simulink model "BD_PAR_SS"  (Simulink 10.3)
settings: Solver=ode1  StartTime=0.0  StopTime=max(cyc_mph(:,1))  FixedStep=1  MaxStep=1  RelTol=1e-3  AbsTol=1e-3
undefined symbols (not defined in the file): acc_elec_eff, acc_elec_pwr, acc_mech_eff, amb_tmp, cs_charge_deplete_bool, cs_electric_decel_spd, cs_electric_launch_spd_hi, cs_electric_launch_spd_lo, cs_hi_soc, cs_lo_soc, cs_off_trq_frac, cyc_avg_time, cyc_cargo_mass, cyc_elevation_init, cyc_filter_bool, cyc_grade, cyc_mph, ess_module_num, ess_on, ess_voc, ex_calc, ex_cat_co_frac, ex_cat_ext_cp, ex_cat_ext_emisv, ex_cat_ext_init_tmp, ex_cat_ext_mass, ex_cat_ext_sarea, ex_cat_hc_frac, ex_cat_i2p_th_cond, ex_cat_i2x_emisv, ex_cat_i2x_th_cond, ex_cat_int_cp, ex_cat_int_init_tmp, ex_cat_int_mass, ex_cat_int_sarea, ex_cat_lim, ex_cat_m2i_th_cond, ex_cat_m2i_tmp, ex_cat_m2p_emisv, ex_cat_mon_cp, ex_cat_mon_init_tmp, ex_cat_mon_mass, ex_cat_mon_sarea, ex_cat_monf_sarea, ex_cat_moni_sarea, ex_cat_nox_frac, ex_cat_p2x_th_cond, ex_cat_pcm_ecp, ex_cat_pcm_mass, ex_cat_pcm_tmp, ex_cat_pipe_cp, ex_cat_pipe_emisv, ex_cat_pipe_init_tmp, ex_cat_pipe_mass, ex_cat_pipe_sarea, ex_cat_pm_frac, ex_cat_tmp_range, ex_gas_cp, ex_manif_cp, ex_manif_emisv ... (+73)
libraries: lib_controls x6, lib_vehicle x3, lib_accessory x2, lib_interactive x1, lib_energy_storage x1, lib_fuel_converter x1
(part 3 of 6)

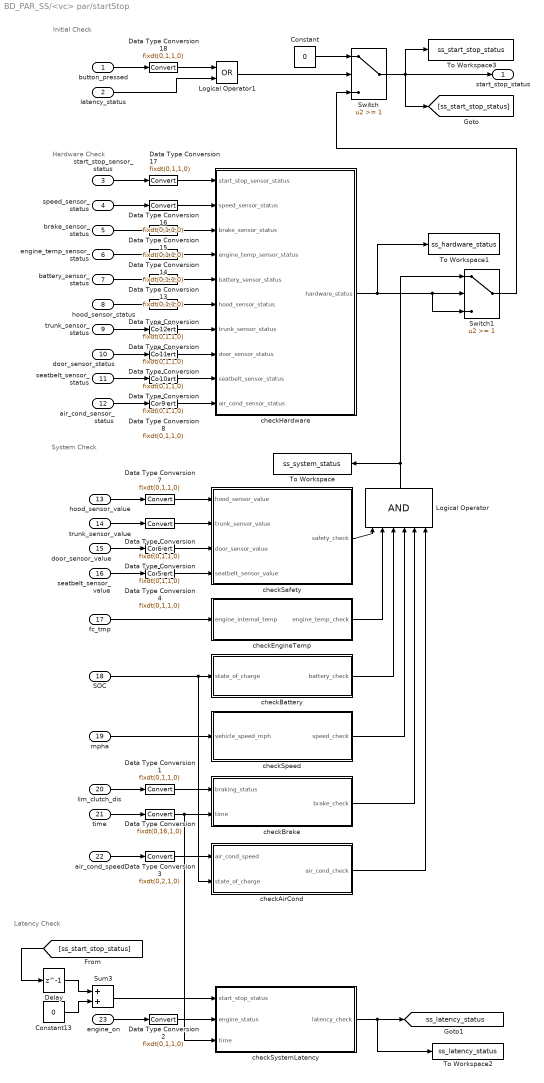
== system BD_PAR_SS/<vc> par/startStop ==
  note: Initial Check
  note: Hardware Check
  note: Latency Check
  note: System Check
  button_pressed : Inport
  latency_status : Inport  Port=2
  start_stop_sensor_status : Inport  Port=3
  speed_sensor_status : Inport  Port=4
  brake_sensor_status : Inport  Port=5
  engine_temp_sensor_status : Inport  Port=6
  battery_sensor_status : Inport  Port=7
  hood_sensor_status : Inport  Port=8
  trunk_sensor_status : Inport  Port=9
  door_sensor_status : Inport  Port=10
  seatbelt_sensor_status : Inport  Port=11
  air_cond_sensor_status : Inport  Port=12
  hood_sensor_value : Inport  Port=13
  trunk_sensor_value : Inport  Port=14
  door_sensor_value : Inport  Port=15
  seatbelt_sensor_value : Inport  Port=16
  fc_tmp : Inport  Port=17
  SOC : Inport  Port=18
  mpha : Inport  Port=19
  lim_clutch_dis : Inport  Port=20
  time : Inport  Port=21
  air_cond_speed : Inport  Port=22
  engine_on : Inport  Port=23
  Constant : Constant  Value=0  OutDataTypeStr=fixdt(0,1,1,0)
  Constant13 : Constant  Value=0  OutDataTypeStr=fixdt(0,1,1,0)
  Data Type Conversion : DataTypeConversion  OutDataTypeStr=fixdt(0,16,1,0)
  Data Type Conversion{1..2,4..18} (17 alike) : DataTypeConversion  OutDataTypeStr=fixdt(0,1,1,0)
  Data Type Conversion3 : DataTypeConversion  OutDataTypeStr=fixdt(0,2,1,0)
  Delay : Delay  DelayLength=1  InitialCondition=0
  Logical Operator : Logic  Inputs=6  AllPortsSameDT=off  OutDataTypeStr=fixdt(0,1,1,0)
  Logical Operator1 : Logic  Operator=OR  AllPortsSameDT=off  OutDataTypeStr=fixdt(0,1,1,0)
  Sum3 : Sum  OutDataTypeStr=fixdt(0,1,1,0)
  Switch : Switch  Threshold=1  OutDataTypeStr=fixdt(0,1,1,0)
  Switch1 : Switch  Threshold=1  OutDataTypeStr=fixdt(0,1,1,0)
  To Workspace : ToWorkspace  VariableName=ss_system_status  SampleTime=-1
  To Workspace1 : ToWorkspace  VariableName=ss_hardware_status  SampleTime=-1
  To Workspace2 : ToWorkspace  VariableName=ss_latency_status  SampleTime=-1
  To Workspace3 : ToWorkspace  VariableName=ss_start_stop_status  SampleTime=-1
  checkAirCond : Subsystem
  checkBattery : Subsystem
  checkBrake : Subsystem
  checkEngineTemp : Subsystem
  checkHardware : Subsystem
  checkSafety : Subsystem
  checkSpeed : Subsystem
  checkSystemLatency : Subsystem
  start_stop_status : Outport
  tag scope: ss_latency_status=global
  wires:
  engine_temp_sensor_status/1 -> Data Type Conversion14/1
  speed_sensor_status/1 -> Data Type Conversion16/1
  Switch/1 -> [ss_start_stop_status], start_stop_status/1, To Workspace3/1
  trunk_sensor_status/1 -> Data Type Conversion11/1
  hood_sensor_status/1 -> Data Type Conversion12/1
  brake_sensor_status/1 -> Data Type Conversion15/1
  battery_sensor_status/1 -> Data Type Conversion13/1
  door_sensor_status/1 -> Data Type Conversion10/1
  seatbelt_sensor_status/1 -> Data Type Conversion9/1
  air_cond_sensor_status/1 -> Data Type Conversion8/1
  button_pressed/1 -> Data Type Conversion18/1
  latency_status/1 -> Logical Operator1/2
  Logical Operator1/1 -> Switch/2
  start_stop_sensor_status/1 -> Data Type Conversion17/1
  checkHardware/1(hardware_status) -> Switch1/2, Switch1/3, To Workspace1/1
  hood_sensor_value/1 -> Data Type Conversion7/1
  trunk_sensor_value/1 -> Data Type Conversion6/1
  door_sensor_value/1 -> Data Type Conversion5/1
  seatbelt_sensor_value/1 -> Data Type Conversion4/1
  fc_tmp/1 -> checkEngineTemp/1(engine_internal_temp)
  SOC/1 -> checkAirCond/2(state_of_charge), checkBattery/1(state_of_charge)
  mpha/1 -> checkSpeed/1(vehicle_speed_mph)
  air_cond_speed/1 -> Data Type Conversion3/1
  time/1 -> Data Type Conversion/1
  lim_clutch_dis/1 -> Data Type Conversion1/1
  checkSafety/1(safety_check) -> Logical Operator/1
  checkEngineTemp/1(engine_temp_check) -> Logical Operator/2
  checkBattery/1(battery_check) -> Logical Operator/3
  checkSpeed/1(speed_check) -> Logical Operator/4
  checkBrake/1(brake_check) -> Logical Operator/5
  checkAirCond/1(air_cond_check) -> Logical Operator/6
  Logical Operator/1 -> Switch1/1, To Workspace/1
  Constant/1 -> Switch/1
  Switch1/1 -> Switch/3
  engine_on/1 -> Data Type Conversion2/1
  checkSystemLatency/1(latency_check) -> [ss_latency_status], To Workspace2/1
  Sum3/1 -> checkSystemLatency/1(start_stop_status)
  [ss_start_stop_status] -> Delay/1
  Data Type Conversion/1 -> checkSystemLatency/3(time), checkBrake/2(time)
  Data Type Conversion1/1 -> checkBrake/1(braking_status)
  Data Type Conversion2/1 -> checkSystemLatency/2(engine_status)
  Data Type Conversion3/1 -> checkAirCond/1(air_cond_speed)
  Constant13/1 -> Sum3/2
  Delay/1 -> Sum3/1
  Data Type Conversion4/1 -> checkSafety/4(seatbelt_sensor_value)
  Data Type Conversion5/1 -> checkSafety/3(door_sensor_value)
  Data Type Conversion6/1 -> checkSafety/2(trunk_sensor_value)
  Data Type Conversion7/1 -> checkSafety/1(hood_sensor_value)
  Data Type Conversion8/1 -> checkHardware/10(air_cond_sensor_status)
  Data Type Conversion9/1 -> checkHardware/9(seatbelt_sensor_status)
  Data Type Conversion10/1 -> checkHardware/8(door_sensor_status)
  Data Type Conversion11/1 -> checkHardware/7(trunk_sensor_status)
  Data Type Conversion14/1 -> checkHardware/4(engine_temp_sensor_status)
  Data Type Conversion15/1 -> checkHardware/3(brake_sensor_status)
  Data Type Conversion13/1 -> checkHardware/5(battery_sensor_status)
  Data Type Conversion12/1 -> checkHardware/6(hood_sensor_status)
  Data Type Conversion16/1 -> checkHardware/2(speed_sensor_status)
  Data Type Conversion17/1 -> checkHardware/1(start_stop_sensor_status)
  Data Type Conversion18/1 -> Logical Operator1/1

== system BD_PAR_SS/NOTES/NOTES ==
  note: ADVISOR 2.0.2 10/7/98
      | Copyright 1998-2003  MRI, NREL.
      | All rights reserved
      |
      |  Notice:  This computer software was
      |  prepared by NREL/MRI, and hereinafter the Contractor,
      | under Contract No. DE-AC36-83CH10093 with
      | the Department of Energy (DOE).  All rights
      | in the computer software are reserved by DOE
      | on behalf of the United States Government and
      | the Contractor as provided in the contract.
      | You are authorized to use this computer software
      | for Governmental purposes but it is not to be
      | released or distributed to the public.  NEITHER
      | THE GOVERNMENT NOR THE CONTRACTOR MAKES ANY
      | WARRANTY, EXPRESS OR IMPLIED, OR ASSUMES ANY
      | LIABILITY FOR THE USE OF THIS SOFTWARE.
      | This notice including this sentence must
      | appear on any copies of this computer software.

== system BD_PAR_SS/clutch <cl>/help ==

== system BD_PAR_SS/drive cycle <cyc>/Block NOTES ==
  note: This block determines the speed required of the vehicle.  If cyc_filter_bool
      | is true, a centered-in-time average of the trace, with backlash, is required of
      | the vehicle.  This may be useful to smooth out jumps in the trace.  Otherwise,
      | the trace, exactly as published, is required of the vehicle.
      | This block also determines the roadway grade of the cycle and the
      | elevation as a function of the distance travelelled

== system BD_PAR_SS/drive cycle <cyc>/ambient pressure calc (atm) ==
  elevation : Inport
  Gain1 : Gain  Gain=-1  SaturateOnIntegerOverflow=on  OutDataTypeStr=Inherit: Same as input  ParamDataTypeStr=Inherit: Same as input
  Height Scale Factor (1/m) : Constant  Value=1.16546e-4
  Math Function : Math  SignedPower=on  SaturateOnIntegerOverflow=on
  Product9 : Product  InputSameDT=on  RndMeth=Zero  SaturateOnIntegerOverflow=on  OutDataTypeStr=Inherit: Same as first input
  Out1 : Outport
  wires:
  Math Function/1 -> Out1/1
  Height Scale Factor (1/m)/1 -> Product9/2
  Gain1/1 -> Product9/1
  elevation/1 -> Gain1/1
  Product9/1 -> Math Function/1

== system BD_PAR_SS/drive cycle <cyc>/distance travelled (m) ==
  Block NOTES : Subsystem
      mask Display: disp('Block\nNOTES')
  Integrator : Integrator
  mph-->m/s : Gain  Gain=0.447  SaturateOnIntegerOverflow=on  OutDataTypeStr=Inherit: Same as input  ParamDataTypeStr=Inherit: Same as input
  Out1 : Outport  InitialOutput=0
  wires:
  mph-->m/s/1 -> Integrator/1
  [mpha] -> mph-->m/s/1
  Integrator/1 -> Out1/1

== system BD_PAR_SS/drive cycle <cyc>/repeated cycle grade vs. distance ==
  distance travelled (m) : Inport
  Fcn1 : Fcn  Expr=rem(u[1],period)
  Look-Up Table : Lookup  InputValues=t  Table=y  SaturateOnIntegerOverflow=on
  out_1 : Outport  InitialOutput=0
  wires:
  Look-Up Table/1 -> out_1/1
  Fcn1/1 -> Look-Up Table/1
  distance travelled (m)/1 -> Fcn1/1

== system BD_PAR_SS/drive cycle <cyc>/repeated cycle speed vs. time ==
  Clock : Clock
  Fcn1 : Fcn  Expr=rem(u[1],period)
  Look-Up Table : Lookup  InputValues=t  Table=y  SaturateOnIntegerOverflow=on
  out_1 : Outport  InitialOutput=0
  wires:
  Look-Up Table/1 -> out_1/1
  Clock/1 -> Fcn1/1
  Fcn1/1 -> Look-Up Table/1

== system BD_PAR_SS/drive cycle <cyc>/repeated cycle vehicle cargo mass vs. distance ==
  distance travelled (m) : Inport
  Fcn1 : Fcn  Expr=rem(u[1],period)
  Look-Up Table : Lookup  InputValues=t  Table=y  SaturateOnIntegerOverflow=on
  out_1 : Outport  InitialOutput=0
  wires:
  Look-Up Table/1 -> out_1/1
  Fcn1/1 -> Look-Up Table/1
  distance travelled (m)/1 -> Fcn1/1

== system BD_PAR_SS/drive cycle <cyc>/super-smooth, no-lag trace ==
  Subsystem : Subsystem  mask(Running Average){n=avgtime}
      mask prompts: n "Averaging Time (s)"
      mask help: Running Average
      mask Help: Output is the average of the last (Averaging Time) seconds of input.
      mask Display: disp('Running\nAverage')
  repeated cycle : Subsystem
  out_1 : Outport  InitialOutput=0
  wires:
  repeated cycle/1(out_1) -> Subsystem/1(in_1)
  Subsystem/1(out_1) -> out_1/1

== system BD_PAR_SS/electric acc loads <acc>/Electrical Accessory Loads v2 <acc> ==
  note: Data Logging
  note: Backward-Forward Models
  note: INTERFACE
  "requested electrical Power, out to the driveline (W)" : Inport
  achieved power in from power source (W) : Inport  Port=2
  on/off : Inport  Port=3
  Accessory SDO : Subsystem
  Block NOTES : Subsystem
      mask Display: disp('Block\nNOTES')
  Mux3 : Mux  Inputs=3
  backward model : Subsystem
  forward model : Subsystem
  memory : Memory  InitialCondition=acc_elec_pwr
  "requested electrical Power, in from the power source (W)" : Outport
  "achieved electrical Power, out to the driveline (W)" : Outport  Port=2
  tag scope: acc_elec_pwr_a=global, acc_elec_pwr_est=global, acc_elec_pwr_r=global
  wires:
  [acc_on] -> backward model/2(on/off)
  on/off/1 -> [acc_on]
  memory/1 -> [acc_elec_pwr_est]
  forward model/2(acc_pwr_out) -> memory/1, [acc_elec_pwr_a]
  [acc_elec_pwr_r] -> forward model/2(acc_pwr_in)
  [acc_elec_pwr_est] -> Mux3/3
  [acc_elec_pwr_a] -> Mux3/2
  [acc_elec_pwr_r] -> Mux3/1
  backward model/2(elec_acc_out) -> [acc_elec_pwr_r]
  Mux3/1 -> Accessory SDO/1(data bus)
  forward model/1(pwr_out) -> [driveline_pwr_out_a]
  [powersource_pwr_in_a] -> forward model/1(pwr_in)
  backward model/1(elec_out) -> [powersource_pwr_in_r]
  [driveline_pwr_out_r] -> backward model/1(pwr_in)
  [driveline_pwr_out_a] -> "achieved electrical Power, out to the driveline (W)"/1
  [powersource_pwr_in_r] -> "requested electrical Power, in from the power source (W)"/1
  achieved power in from power source (W)/1 -> [powersource_pwr_in_a]
  "requested electrical Power, out to the driveline (W)"/1 -> [driveline_pwr_out_r]

== system BD_PAR_SS/energy storage <ess>/ess config ==
  power req'd into bus (W) : Inport
  energy storage <ess> : lib_energy_storage/Ess Choices/energy storage <ess>  SystemSampleTime=-1  VariantActivationTime=update diagram  Latency=0  AutoFrameSizeCalculation=off
  power available to bus (W) : Outport
  wires:
  power req'd into bus (W)/1 -> energy storage <ess>/1
  energy storage <ess>/1 -> power available to bus (W)/1

== system BD_PAR_SS/exhaust sys <ex>/Block NOTES ==
  note: This block models the exhaust system of an internal combustion engine (ICE).  Emphasis is on the catalytic converter
      | aftertreatment of emissions.  Since converter performance is tied to operating temperature, the temperature and heat
      | flows of the exhaust gas, converter, and engine manifold/downpipe are predicted.

== system BD_PAR_SS/exhaust sys <ex>/ex gas heat flow ==
  emis cat'd : Inport
  ex gas flow : Inport  Port=2
  Tex,eo : Inport  Port=3
  ex_temp : Inport  Port=4
  Enable : EnablePort  StatesWhenEnabling=reset
  % : Gain  Gain=100  SaturateOnIntegerOverflow=on
  %1 : Gain  Gain=669  SaturateOnIntegerOverflow=on
  %2 : Gain  Gain=121  SaturateOnIntegerOverflow=on
  %3 : Gain  Gain=93+79/3  SaturateOnIntegerOverflow=on
  %5 : Gain  Gain=0  SaturateOnIntegerOverflow=on
  (eo-tp)/exg : Product  Inputs=*/  SaturateOnIntegerOverflow=on
  Block NOTES : Subsystem
      mask Display: disp('Block\nNOTES')
  Demux3 : Demux
  Memory : Memory  InitialCondition=[0 0 0 0]
  Mux17 : Mux
  Mux19 : Mux  Inputs=3
  Qcp5 : Sum  Inputs=+-  SaturateOnIntegerOverflow=on
  Saturation1 : Saturate  UpperLimit=1  LowerLimit=0
  converter : Subsystem
  cp,exg : Gain  Gain=ex_gas_cp/1000  SaturateOnIntegerOverflow=on
  dTcat : Sum  Inputs=++++  SaturateOnIntegerOverflow=on
  h,exg : Fcn  Expr=23*((u/10)^0.8)
  inlet pipe : Subsystem
  "manifold " : Subsystem
  mol_EO/s : Gain  Gain=[1/44.1 1/28 1/46 1/44]  SaturateOnIntegerOverflow=on
  mol_ex/s : Gain  Gain=1/29  SaturateOnIntegerOverflow=on
  tailpipe  emis : Product  SaturateOnIntegerOverflow=on
  Tex,gas : Outport  OutputWhenDisabled=reset  InitialOutput=amb_tmp
  Qcat : Outport  Port=2  OutputWhenDisabled=reset  InitialOutput=0
  Qex : Outport  Port=3  OutputWhenDisabled=reset  InitialOutput=0
  wires:
  Memory/1 -> mol_EO/s/1
  emis cat'd/1 -> Memory/1
  ex gas flow/1 -> cp,exg/1, h,exg/1, mol_ex/s/1
  "manifold "/1(Texgo) -> inlet pipe/3(Texgi)
  %2/1 -> dTcat/3
  %3/1 -> dTcat/2
  %1/1 -> dTcat/1
  dTcat/1 -> tailpipe  emis/1
  tailpipe  emis/1 -> Qcat/1
  Mux19/1 -> Tex,gas/1
  Mux17/1 -> Qex/1
  [Tgmo] -> Mux19/3
  [Tgpo] -> Mux19/2
  converter/1(Texgo) -> Mux19/1
  converter/2(Qcm2g) -> Mux17/1
  converter/3(Qci2g) -> Mux17/2
  [Qp2g] -> Mux17/3
  [Qma2g] -> Mux17/4
  %5/1 -> dTcat/4
  inlet pipe/1(Texgo) -> converter/3(Texgi)
  Demux3/2 -> Qcp5/1
  Demux3/3 -> Qcp5/2, %2/1
  Demux3/1 -> %1/1
  Qcp5/1 -> %3/1
  Demux3/4 -> %5/1
  Saturation1/1 -> %/1
  mol_ex/s/1 -> (eo-tp)/exg/2
  mol_EO/s/1 -> (eo-tp)/exg/1
  (eo-tp)/exg/1 -> Saturation1/1
  Tex,eo/1 -> "manifold "/3(Texgi)
  ex_temp/1 -> inlet pipe/4(Tex), converter/4(Tex), "manifold "/4(Tex)
  cp,exg/1 -> inlet pipe/2(Cexg), tailpipe  emis/2, converter/2(Cexg), "manifold "/2(Cexg)
  h,exg/1 -> inlet pipe/1(h,exg), converter/1(h,exg), "manifold "/1(h,exg)
  %/1 -> Demux3/1

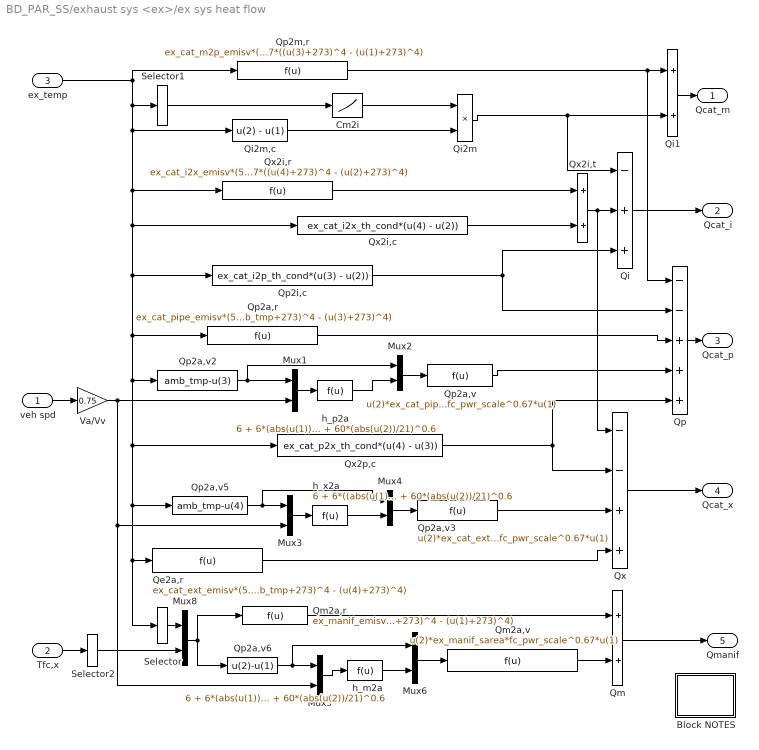
== system BD_PAR_SS/exhaust sys <ex>/ex sys heat flow ==
  veh spd : Inport
  Tfc,x : Inport  Port=2
  ex_temp : Inport  Port=3
  Block NOTES : Subsystem
      mask Display: disp('Block\nNOTES')
  Cm2i : Lookup  InputValues=ex_cat_m2i_tmp  Table=ex_cat_m2i_th_cond  SaturateOnIntegerOverflow=on
  Mux{1..6,8} (7 alike) : Mux  Inputs=2
  Qe2a,r : Fcn  Expr=ex_cat_ext_emisv*(5.67e-8)*ex_cat_ext_sarea*fc_pwr_scale^0.67*((amb_tmp+273)^4 - (u(4)+273)^4)
  Qi : Sum  Inputs=-++  SaturateOnIntegerOverflow=on
  Qi1 : Sum  SaturateOnIntegerOverflow=on
  Qi2m : Product  SaturateOnIntegerOverflow=on
  Qi2m,c : Fcn  Expr=u(2) - u(1)
  Qm : Sum  SaturateOnIntegerOverflow=on
  Qm2a,r : Fcn  Expr=ex_manif_emisv*(5.67e-8)*ex_manif_sarea*fc_pwr_scale^0.67*((u(2)+273)^4 - (u(1)+273)^4)
  Qm2a,v : Fcn  Expr=u(2)*ex_manif_sarea*fc_pwr_scale^0.67*u(1)
  Qp : Sum  Inputs=--+++  SaturateOnIntegerOverflow=on
  Qp2a,r : Fcn  Expr=ex_cat_pipe_emisv*(5.67e-8)*ex_cat_pipe_sarea*fc_pwr_scale^0.67*((amb_tmp+273)^4 - (u(3)+273)^4)
  Qp2a,v : Fcn  Expr=u(2)*ex_cat_pipe_sarea*fc_pwr_scale^0.67*u(1)
  Qp2a,v2 : Fcn  Expr=amb_tmp-u(3)
  Qp2a,v3 : Fcn  Expr=u(2)*ex_cat_ext_sarea*fc_pwr_scale^0.67*u(1)
  Qp2a,v5 : Fcn  Expr=amb_tmp-u(4)
  Qp2a,v6 : Fcn  Expr=u(2)-u(1)
  Qp2i,c : Fcn  Expr=ex_cat_i2p_th_cond*(u(3) - u(2))
  Qp2m,r : Fcn  Expr=ex_cat_m2p_emisv*(5.67e-8)*ex_cat_monf_sarea*fc_pwr_scale^0.67*((u(3)+273)^4 - (u(1)+273)^4)
  Qx : Sum  Inputs=--++  SaturateOnIntegerOverflow=on
  Qx2i,c : Fcn  Expr=ex_cat_i2x_th_cond*(u(4) - u(2))
  Qx2i,r : Fcn  Expr=ex_cat_i2x_emisv*(5.67e-8)*ex_cat_int_sarea*fc_pwr_scale^0.67*((u(4)+273)^4 - (u(2)+273)^4)
  Qx2i,t : Sum  SaturateOnIntegerOverflow=on
  Qx2p,c : Fcn  Expr=ex_cat_p2x_th_cond*(u(4) - u(3))
  Selector : Selector  InputPortWidth=5  IndexOptions=Index vector (dialog)  Indices=5  OutputSizes=1
  Selector1 : Selector  InputPortWidth=5  IndexOptions=Index vector (dialog)  Indices=[2]  OutputSizes=1
  Selector2 : Selector  InputPortWidth=4  IndexOptions=Index vector (dialog)  Indices=3  OutputSizes=1
  Va/Vv : Gain  Gain=0.75  SaturateOnIntegerOverflow=on
  h_m2a : Fcn  Expr=6 + 6*(abs(u(1))/1000)^0.3 + 60*(abs(u(2))/21)^0.6
  h_p2a : Fcn  Expr=6 + 6*(abs(u(1))/1000)^0.3 + 60*(abs(u(2))/21)^0.6
  h_x2a : Fcn  Expr=6 + 6*((abs(u(1))/1000))^0.3 + 60*(abs(u(2))/21)^0.6
  Qcat_m : Outport
  Qcat_i : Outport  Port=2
  Qcat_p : Outport  Port=3
  Qcat_x : Outport  Port=4
  Qmanif : Outport  Port=5
  wires:
  ex_temp/1 -> Qx2i,c/1, Qx2i,r/1, Qp2m,r/1, Selector1/1, Qi2m,c/1, Qp2i,c/1, Qp2a,r/1, Qp2a,v2/1, Qx2p,c/1, Qp2a,v5/1, Qe2a,r/1, Selector/1
  Qi/1 -> Qcat_i/1
  Qp/1 -> Qcat_p/1
  Mux1/1 -> h_p2a/1
  Qp2a,v2/1 -> Mux1/1, Mux2/1
  Mux4/1 -> Qp2a,v3/1
  Qx/1 -> Qcat_x/1
  Qi1/1 -> Qcat_m/1
  Qx2i,c/1 -> Qx2i,t/2
  Qi2m,c/1 -> Qi2m/2
  Qi2m/1 -> Qi1/2, Qi/1
  Selector1/1 -> Cm2i/1
  Cm2i/1 -> Qi2m/1
  Qp2i,c/1 -> Qi/3, Qp/2
  Qp2m,r/1 -> Qi1/1, Qp/1
  Qp2a,r/1 -> Qp/3
  Qp2a,v/1 -> Qp/4
  Qx2i,r/1 -> Qx2i,t/1
  Qx2i,t/1 -> Qi/2, Qx/1
  Qp2a,v3/1 -> Qx/3
  Mux3/1 -> h_x2a/1
  Qp2a,v5/1 -> Mux3/1, Mux4/1
  h_x2a/1 -> Mux4/2
  Qe2a,r/1 -> Qx/4
  Mux2/1 -> Qp2a,v/1
  h_p2a/1 -> Mux2/2
  Qx2p,c/1 -> Qp/5, Qx/2
  Qm2a,v/1 -> Qm/2
  Qm/1 -> Qmanif/1
  Qm2a,r/1 -> Qm/1
  Mux6/1 -> Qm2a,v/1
  Mux5/1 -> h_m2a/1
  Qp2a,v6/1 -> Mux5/1, Mux6/1
  Selector/1 -> Mux8/1
  Mux8/1 -> Qm2a,r/1, Qp2a,v6/1
  h_m2a/1 -> Mux6/2
  Tfc,x/1 -> Selector2/1
  Selector2/1 -> Mux8/2
  veh spd/1 -> Va/Vv/1
  Va/Vv/1 -> Mux3/2, Mux5/2, Mux1/2

== system BD_PAR_SS/exhaust sys <ex>/help ==

== system BD_PAR_SS/exhaust sys <ex>/removal efficiencies ==
  gas_flow (g/s) : Inport
  Ex Gas T (C) : Inport  Port=2
  O2_exh (g/s) : Inport  Port=3
  emis Engine Out (g/s) : Inport  Port=4
  Ex Cat T (C) : Inport  Port=5
  =1: use ORNL data =0: use base ADVISOR : Constant  Value=ex_ornl_bool
  Switch : Switch  Threshold=eps  SaturateOnIntegerOverflow=on  InputSameDT=on
  cat in  gas tmp : Selector  InputPortWidth=3  IndexOptions=Index vector (dialog)  Indices=2  OutputSizes=1
  ex_ornl_bool=0 : Logic  Operator=NOT
  removal efficiencies (base ADVISOR) : Subsystem  TreatAsAtomicUnit=on
  removal efficiencies ORNL : Subsystem  TreatAsAtomicUnit=on
  removal effs : Outport  OutputWhenDisabled=reset  InitialOutput=0
  wires:
  removal efficiencies (base ADVISOR)/1(removal effs) -> Switch/1
  removal efficiencies ORNL/1(removal effs) -> Switch/3
  =1: use ORNL data =0: use base ADVISOR/1 -> removal efficiencies ORNL/Enable, ex_ornl_bool=0/1
  O2_exh (g/s)/1 -> removal efficiencies ORNL/3(O2_exh (g/s))
  gas_flow (g/s)/1 -> removal efficiencies ORNL/1(gas_flow (g/s))
  emis Engine Out (g/s)/1 -> removal efficiencies ORNL/4(emis Engine Out (g/s))
  cat in  gas tmp/1 -> removal efficiencies ORNL/2(Ex Gas T (C))
  Ex Gas T (C)/1 -> cat in  gas tmp/1
  Switch/1 -> removal effs/1
  Ex Cat T (C)/1 -> removal efficiencies ORNL/5(Ex Cat T (C)), removal efficiencies (base ADVISOR)/1(Ex Cat T (C))
  ex_ornl_bool=0/1 -> Switch/2, removal efficiencies (base ADVISOR)/Enable

== system BD_PAR_SS/final drive <fd>/Block NOTES ==
  note: The inertia torque is the input torque required to accelerate the
      | final drive's inertia as measured on the input side.
  note: The loss torque is zero when the gears are not turning,
      | and is applied at the input side of the gear reduction.
  note: This final drive model includes loss data, rotational inertia, and a gear reduction.

== system BD_PAR_SS/final drive <fd>/effect of inertia (Nm) ==
  note: The inertia torque is the input torque required to accelerate the
      | final drive's inertia as measured on the input side.
  fd input speed (rad/s) : Inport
  Gain : Gain  Gain=fd_inertia  SaturateOnIntegerOverflow=on
  d/dt : Derivative
  drag torque (Nm) : Outport  InitialOutput=0
  wires:
  fd input speed (rad/s)/1 -> d/dt/1
  d/dt/1 -> Gain/1
  Gain/1 -> drag torque (Nm)/1

== system BD_PAR_SS/final drive <fd>/help ==

== system BD_PAR_SS/final drive <fd>/loss (Nm) ==
  note: The loss torque is zero when the gears are not turning,
      | and is applied at the input side of the gear reduction.
  fd output speed (rad/s) : Inport
  Constant : Constant  Value=0
  Switch : Switch  Threshold=eps  SaturateOnIntegerOverflow=on  InputSameDT=on
  final drive loss torque (Nm) : Constant  Value=fd_loss
  drag torque (Nm) : Outport  InitialOutput=0
  wires:
  Constant/1 -> Switch/3
  fd output speed (rad/s)/1 -> Switch/2
  Switch/1 -> drag torque (Nm)/1
  final drive loss torque (Nm)/1 -> Switch/1

== system BD_PAR_SS/fuel converter  <fc>/Block NOTES ==
  note: This block models the internal combustion engine, and includes inertia effects,
      | performance limits, accessory loads, and temperature transient effects on fuel
      | use, engine-out emissions, and catalyst efficiency.  There are 'leads' to the
      | engine controller here, which controller determines whether the engine is on.

== system BD_PAR_SS/fuel converter  <fc>/engine controller interface ==
  fc_spd_out_r : Inport
  spd command : Outport
  tag scope: fc_spd_out_r=global
  wires:
  [spd_command] -> spd command/1
  fc_spd_out_r/1 -> [fc_spd_out_r]

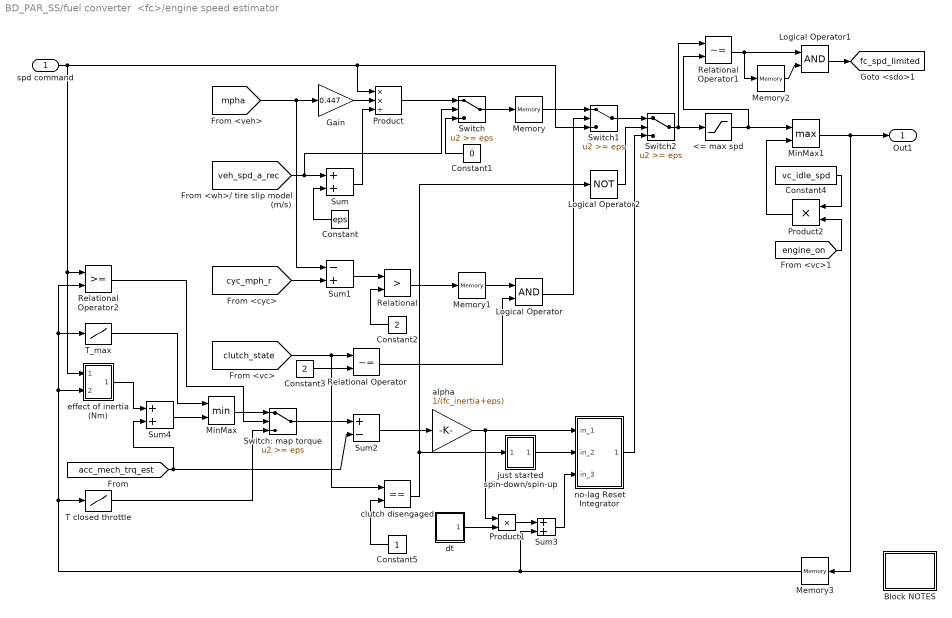
== system BD_PAR_SS/fuel converter  <fc>/engine speed estimator ==
  spd command : Inport
  <= max spd : Saturate  UpperLimit=max(fc_map_spd)*fc_spd_scale  LowerLimit=-inf
  Block NOTES : Subsystem
      mask Display: disp('Block\nNOTES')
  Constant : Constant  Value=eps
  Constant1 : Constant  Value=0
  Constant2 : Constant  Value=2
  Constant3 : Constant  Value=2
  Constant4 : Constant  Value=vc_idle_spd
  Constant5 : Constant
  Gain : Gain  Gain=0.447  SaturateOnIntegerOverflow=on  OutDataTypeStr=Inherit: Same as input  ParamDataTypeStr=Inherit: Same as input
  Logical Operator : Logic
  Logical Operator1 : Logic
  Logical Operator2 : Logic  Operator=NOT  Inputs=1
  Memory : Memory  InitialCondition=cyc_mph(1,2)*0.447/wh_radius*fd_ratio*gb_ratio(gb_num_init)
  Memory1 : Memory
  Memory2 : Memory
  Memory3 : Memory  InitialCondition=cyc_mph(1,2)*0.447/wh_radius*fd_ratio*max(gb_ratio)
  MinMax : MinMax  Inputs=2  InputSameDT=on  SaturateOnIntegerOverflow=on
  MinMax1 : MinMax  Function=max  Inputs=2  InputSameDT=on  SaturateOnIntegerOverflow=on
  Product : Product  Inputs=**/  InputSameDT=on  RndMeth=Zero  SaturateOnIntegerOverflow=on  OutDataTypeStr=Inherit: Same as first input
  Product1 : Product  InputSameDT=on  RndMeth=Zero  SaturateOnIntegerOverflow=on  OutDataTypeStr=Inherit: Same as first input
  Product2 : Product  InputSameDT=on  RndMeth=Zero  SaturateOnIntegerOverflow=on  OutDataTypeStr=Inherit: Same as first input
  Relational : RelationalOperator  Operator=>  RndMeth=Nearest  InputSameDT=on
  Relational Operator : RelationalOperator  Operator=~=  RndMeth=Nearest  InputSameDT=on
  Relational Operator1 : RelationalOperator  Operator=~=  RndMeth=Nearest  InputSameDT=on
  Relational Operator2 : RelationalOperator  RndMeth=Nearest  InputSameDT=on
  Sum : Sum  InputSameDT=on  SaturateOnIntegerOverflow=on  OutDataTypeStr=Inherit: Same as first input
  Sum1 : Sum  Inputs=-+  InputSameDT=on  SaturateOnIntegerOverflow=on  OutDataTypeStr=Inherit: Same as first input
  Sum2 : Sum  Inputs=+-  InputSameDT=on  SaturateOnIntegerOverflow=on  OutDataTypeStr=Inherit: Same as first input
  Sum3 : Sum  InputSameDT=on  SaturateOnIntegerOverflow=on  OutDataTypeStr=Inherit: Same as first input
  Sum4 : Sum  InputSameDT=on  SaturateOnIntegerOverflow=on  OutDataTypeStr=Inherit: Same as first input
  Switch : Switch  Threshold=eps  SaturateOnIntegerOverflow=on  InputSameDT=on
  Switch1 : Switch  Threshold=eps  SaturateOnIntegerOverflow=on  InputSameDT=on
  Switch2 : Switch  Threshold=eps  SaturateOnIntegerOverflow=on  InputSameDT=on
  Switch: map torque : Switch  Threshold=eps  SaturateOnIntegerOverflow=on  InputSameDT=on
  T closed throttle : Lookup  InputValues=fc_map_spd*fc_spd_scale  Table=fc_ct_trq*fc_trq_scale  SaturateOnIntegerOverflow=on
  T_max : Lookup  InputValues=fc_map_spd*fc_spd_scale  Table=fc_max_trq*fc_trq_scale  SaturateOnIntegerOverflow=on
  alpha : Gain  Gain=1/(fc_inertia+eps)  SaturateOnIntegerOverflow=on  OutDataTypeStr=Inherit: Same as input  ParamDataTypeStr=Inherit: Same as input
  clutch disengaged : RelationalOperator  Operator===  RndMeth=Nearest  InputSameDT=on
  dt : Subsystem
  effect of inertia (Nm) : Subsystem
  just started spin-down/spin-up : Subsystem
  no-lag Reset Integrator : Subsystem  mask(No-lag Reset Integrator){initval=vc_idle_spd}
      mask prompts: initval "Initial Value"
      mask help: No-lag Reset Integrator
      mask Help: Integrates first input using Euler technique.\nAt the time step that input 2 <> zero,\noutput is reset to input 3.
      mask Display: disp('1/s\nw/ reset\nno lag')
  Out1 : Outport
  tag scope: fc_spd_limited=global
  wires:
  [acc_mech_trq_est] -> Sum2/2, Sum4/2
  Product/1 -> Switch/1
  [veh_spd_a_rec] -> Sum/1, Switch/2
  Constant1/1 -> Switch/3
  Memory/1 -> Switch1/1
  Constant/1 -> Sum/2
  [cyc_mph_r] -> Sum1/2
  [mpha] -> Gain/1, Sum1/1
  Constant2/1 -> Relational/2
  Sum1/1 -> Relational/1
  Relational/1 -> Memory1/1
  Switch/1 -> Memory/1
  Gain/1 -> Product/2
  Sum/1 -> Product/3
  Relational Operator/1 -> Logical Operator/2
  Memory1/1 -> Logical Operator/1
  Constant3/1 -> Relational Operator/2
  Sum2/1 -> alpha/1
  dt/1(out_1) -> Product1/2
  Product1/1 -> Sum3/1
  alpha/1 -> Product1/1, no-lag Reset Integrator/1(in_1)
  Constant5/1 -> clutch disengaged/2
  Switch1/1 -> Switch2/1
  clutch disengaged/1 -> Logical Operator2/1, just started spin-down/spin-up/1(state)
  [clutch_state] -> Relational Operator/1, clutch disengaged/1
  Memory3/1 -> Sum3/2, Relational Operator2/2, T_max/1, effect of inertia (Nm)/2(prev spd), T closed throttle/1
  <= max spd/1 -> Relational Operator1/2, MinMax1/1
  [engine_on] -> Product2/2
  Constant4/1 -> Product2/1
  MinMax1/1 -> Out1/1, Memory3/1
  Product2/1 -> MinMax1/2
  Switch2/1 -> <= max spd/1, Relational Operator1/1
  Memory2/1 -> Logical Operator1/2
  Logical Operator1/1 -> [fc_spd_limited]
  Relational Operator1/1 -> Logical Operator1/1, Memory2/1
  Switch: map torque/1 -> Sum2/1
  Relational Operator2/1 -> Switch: map torque/2
  T closed throttle/1 -> Switch: map torque/3
  MinMax/1 -> Switch: map torque/1
  T_max/1 -> MinMax/1
  Sum4/1 -> MinMax/2
  effect of inertia (Nm)/1((Nm)) -> Sum4/1
  spd command/1 -> Relational Operator2/1, effect of inertia (Nm)/1(req'd spd (rad/s)), Switch1/3, Product/1
  Logical Operator2/1 -> Switch2/2
  Logical Operator/1 -> Switch1/2
  no-lag Reset Integrator/1(out_1) -> Switch2/3
  just started spin-down/spin-up/1(trigger) -> no-lag Reset Integrator/2(in_2)
  Sum3/1 -> no-lag Reset Integrator/3(in_3)

== system BD_PAR_SS/fuel converter  <fc>/engine torque ==
  fc_trq_out_r : Inport
  spd command : Inport  Port=2
  engine spd : Inport  Port=3
  Block NOTES : Subsystem
      mask Display: disp('Block\nNOTES')
  Constant1 : Constant  Value=0
  Constant3 : Constant
  Logical Operator : Logic  Operator=OR
  MinMax : MinMax  Inputs=2  InputSameDT=on  SaturateOnIntegerOverflow=on
  MinMax1 : MinMax  Function=max  Inputs=2  InputSameDT=on  SaturateOnIntegerOverflow=on
  Sum : Sum  InputSameDT=on  SaturateOnIntegerOverflow=on  OutDataTypeStr=Inherit: Same as first input
  Sum1 : Sum  Inputs=+-  InputSameDT=on  SaturateOnIntegerOverflow=on  OutDataTypeStr=Inherit: Same as first input
  Switch : Switch  Threshold=eps  SaturateOnIntegerOverflow=on  InputSameDT=on
  Switch1 : Switch  Threshold=eps  SaturateOnIntegerOverflow=on  InputSameDT=on
  T_closed throttle : Subsystem
  T_max : Subsystem
  clutch not disengaged : RelationalOperator  Operator=~=  RndMeth=Nearest  InputSameDT=on
  effect of inertia (Nm) : Subsystem
  engine commanded not to decelerate : RelationalOperator  Operator=<=  RndMeth=Nearest  InputSameDT=on
  limited : RelationalOperator  Operator=~=  RndMeth=Nearest  InputSameDT=on
  map torque (Nm) : Outport
  torque to shaft (Nm) : Outport  Port=2
  tag scope: fc_trq_limited=global
  wires:
  Constant1/1 -> Switch1/3
  Sum1/1 -> Switch1/1
  Switch1/1 -> torque to shaft (Nm)/1
  [clutch_state] -> clutch not disengaged/1
  Constant3/1 -> clutch not disengaged/2
  engine commanded not to decelerate/1 -> Logical Operator/1
  Sum/1 -> Switch/1
  Logical Operator/1 -> Switch/2
  limited/1 -> [fc_trq_limited]
  MinMax/1 -> MinMax1/1
  T_max/1(T_max) -> MinMax/2
  T_closed throttle/1(T_closed throttle) -> Switch/3, MinMax1/2
  MinMax1/1 -> limited/2, map torque (Nm)/1, Sum1/1
  Switch/1 -> MinMax/1, limited/1
  clutch not disengaged/1 -> Switch1/2, Logical Operator/2
  engine spd/1 -> T_closed throttle/1(w_APU), T_max/1(w_APU), engine commanded not to decelerate/1, effect of inertia (Nm)/1(engine spd (rad/s))
  fc_trq_out_r/1 -> Sum/1
  effect of inertia (Nm)/1((Nm)) -> Sum/2, Sum1/2
  spd command/1 -> engine commanded not to decelerate/2

== system BD_PAR_SS/fuel converter  <fc>/fuel use and EO emis Configurable Subsystem ==
  T (Nm) : Inport
  w (rad/s) : Inport  Port=2
  fuel use and EO emis : lib_fuel_converter/configurable subsystems/fuel use and EO emis  SystemSampleTime=-1  VariantActivationTime=update diagram  Latency=0  AutoFrameSizeCalculation=off
  cumulative fuel  use (gal) : Outport
  "FC ON?, EOem, MFex, Tex, O2ex" : Outport  Port=2
  Vv,Tfc : Outport  Port=3
  wires:
  T (Nm)/1 -> fuel use and EO emis/1
  w (rad/s)/1 -> fuel use and EO emis/2
  fuel use and EO emis/1 -> cumulative fuel  use (gal)/1
  fuel use and EO emis/2 -> "FC ON?, EOem, MFex, Tex, O2ex"/1
  fuel use and EO emis/3 -> Vv,Tfc/1

== system BD_PAR_SS/fuel converter  <fc>/help ==

== system BD_PAR_SS/gearbox <gb>/Block NOTES ==
  note: This is a good assumption, at least for the VW 4-speed manual transaxle of SAE 820741.
      | In the VW transaxle, efficiency is fairly independent of torque and speed at high torques.
  note: Available output torque is estimated assuming that the gearbox efficiency for theavailable input
      | torque andspeed is the same as the gearbox efficiency for the REQUESTED input torque.
  note: The inertia torque is the input torque required to accelerate the
      | final drive's inertia as measured on the input side.
  note: The loss torque is zero when the gears are not turning,
      | and is applied at the input side of the gear reduction.
  note: This gearbox model includes loss data, rotational inertia, and a gear reduction.

== system BD_PAR_SS/gearbox <gb>/Pout/Pin, neglecting inertia ==
  note: Pout/Pin, neglecting inertia, is used to estimate the output torque given the
      | input torque in a very simple forward-facing calculation.
  Tin : Inport
  Tinertia : Inport  Port=2
  Tout : Inport  Port=3
  gear ratio : Inport  Port=4
  Constant1 : Constant  Value=0
  Pout/Pin (neglecting inertia) : Subsystem
      mask Display: disp('/')
  Product : Product  SaturateOnIntegerOverflow=on
  Relational Operator : RelationalOperator  Operator=~=  RndMeth=Nearest  InputSameDT=on
  Saturation : Saturate  UpperLimit=inf  LowerLimit=0
  Switch : Switch  Threshold=eps  SaturateOnIntegerOverflow=on  InputSameDT=on
  Tin-Tinertia : Sum  Inputs=+-  SaturateOnIntegerOverflow=on
  make division bombproof : Subsystem
  Pout/Pin : Outport  InitialOutput=0
  wires:
  gear ratio/1 -> Product/1
  Product/1 -> Pout/Pin (neglecting inertia)/2(in_2)
  Tout/1 -> Pout/Pin (neglecting inertia)/1(in_1)
  Tin-Tinertia/1 -> Relational Operator/1, make division bombproof/1(Tin-Tinertia)
  Saturation/1 -> Pout/Pin/1
  Switch/1 -> Saturation/1
  Relational Operator/1 -> Switch/2
  Pout/Pin (neglecting inertia)/1(out_1) -> Switch/1
  Tin/1 -> Tin-Tinertia/1
  Tinertia/1 -> Tin-Tinertia/2
  make division bombproof/1(Out1) -> Product/2
  Constant1/1 -> Relational Operator/2, Switch/3

== system BD_PAR_SS/gearbox <gb>/effect of inertia (Nm) ==
  note: The inertia torque is the input torque required to accelerate the
      | gearbox's inertia as measured on the input side.
  gb input speed (rad/s) : Inport
  Gain : Gain  Gain=gb_inertia  SaturateOnIntegerOverflow=on
  d/dt : Derivative
  drag torque (Nm) : Outport  InitialOutput=0
  wires:
  gb input speed (rad/s)/1 -> d/dt/1
  d/dt/1 -> Gain/1
  Gain/1 -> drag torque (Nm)/1

== system BD_PAR_SS/gearbox <gb>/gearbox controller interface ==
  T_gb_out : Inport
  w_gb_out : Inport  Port=2
  eta_gb : Inport  Port=3
  gear_ratio : Outport  InitialOutput=0
  shifting : Outport  Port=2  InitialOutput=0
  tag scope: T_gb_out=global, eta_gb=global, w_gb_out=global
  wires:
  [shifting] -> shifting/1
  T_gb_out/1 -> [T_gb_out]
  w_gb_out/1 -> [w_gb_out]
  eta_gb/1 -> [eta_gb]
  [gear_ratio] -> gear_ratio/1

== system BD_PAR_SS/gearbox <gb>/gearing (Nm), (rad/s) ==
  "output shaft torque and speed  (Nm), (rad/s)" : Inport
  gear ratio : Inport  Port=2
  Demux : Demux  Outputs=2
  Fcn1 : Fcn  Expr=1/u
  Product2 : Product  SaturateOnIntegerOverflow=on
  Product3 : Product  SaturateOnIntegerOverflow=on
  input shaft torque (Nm) : Outport  InitialOutput=0
  input shaft speed (rad/s) : Outport  Port=2  InitialOutput=0
  wires:
  Demux/2 -> Product3/1
  Demux/1 -> Product2/1
  gear ratio/1 -> Product3/2, Fcn1/1
  "output shaft torque and speed  (Nm), (rad/s)"/1 -> Demux/1
  Fcn1/1 -> Product2/2
  Product2/1 -> input shaft torque (Nm)/1
  Product3/1 -> input shaft speed (rad/s)/1

== system BD_PAR_SS/gearbox <gb>/gearing (Nm), (rad/s)1 ==
  input shaft torque (Nm) : Inport
  input shaft speed (rad/s) : Inport  Port=2
  gear ratio : Inport  Port=3
  Fcn1 : Fcn  Expr=1/u
  Product2 : Product  SaturateOnIntegerOverflow=on
  Product3 : Product  SaturateOnIntegerOverflow=on
  output shaft torque (Nm) : Outport  InitialOutput=0
  output shaft speed (rad/s) : Outport  Port=2  InitialOutput=0
  wires:
  input shaft speed (rad/s)/1 -> Product3/2
  input shaft torque (Nm)/1 -> Product2/1
  Product2/1 -> output shaft torque (Nm)/1
  Product3/1 -> output shaft speed (rad/s)/1
  gear ratio/1 -> Fcn1/1, Product2/2
  Fcn1/1 -> Product3/1

== system BD_PAR_SS/gearbox <gb>/help ==

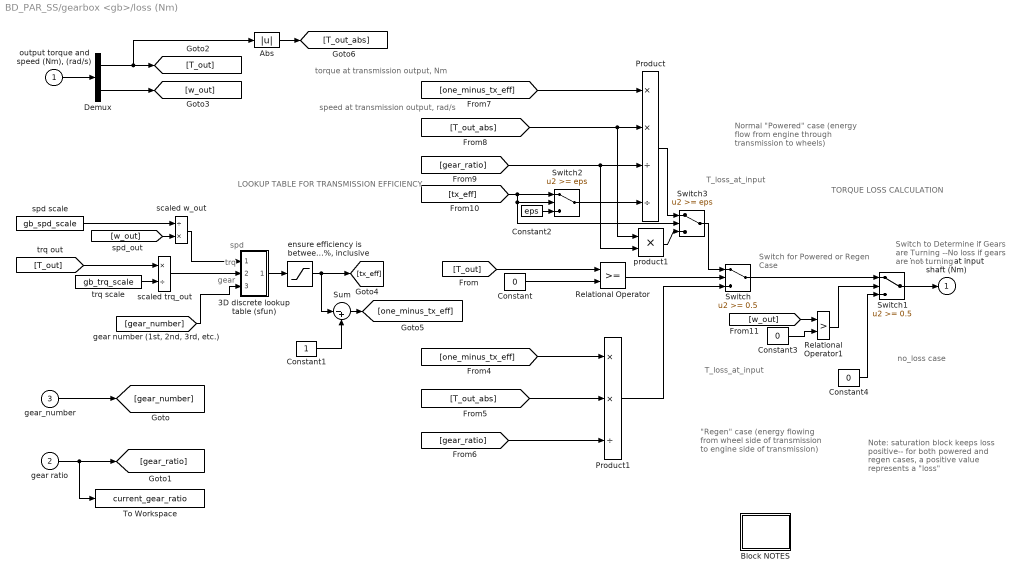
== system BD_PAR_SS/gearbox <gb>/loss (Nm) ==
  note: TORQUE LOSS CALCULATION
  note: gear
  note: trq
  note: spd
  note: torque at transmission output, Nm
  note: speed at transmission output, rad/s
  note: no_loss case
  note: Note: saturation block keeps
      | loss positive-- for both powered
      | and regen cases, a
      | positive value represents a "loss"
  note: Switch for Powered
      |  or Regen Case
  note: Switch to Determine
      | if Gears are Turning
      | --No loss if gears
      | are not turning
  note: Normal "Powered" case
      | (energy flow from engine
      | through transmission to wheels)
  note: T_loss_at_input
  note: "Regen" case
      | (energy flowing from
      | wheel side of transmission
      | to engine side of transmission)
  note: T_loss_at_input
  note: LOOKUP TABLE FOR TRANSMISSION EFFICIENCY
  "output torque and speed (Nm), (rad/s)" : Inport
  gear ratio : Inport  Port=2
  gear_number : Inport  Port=3
  3D discrete lookup table (sfun) : Subsystem  mask{tx_map_spd=tx_map_spd, tx_map_trq=tx_map_trq, tx_eff_map=tx_eff_map}
      mask prompts: tx_map_spd "Row Lookup"; tx_map_trq "Column Lookup"; tx_eff_map "Lookup Matrix"
  Abs : Abs  SaturateOnIntegerOverflow=on
  Block NOTES : Subsystem
      mask Display: disp('Block\nNOTES')
  Constant : Constant  Value=0
  Constant1 : Constant
  Constant2 : Constant  Value=eps
  Constant3 : Constant  Value=0
  Constant4 : Constant  Value=0
  Demux : Demux  Outputs=2
  Product : Product  Inputs=**//  SaturateOnIntegerOverflow=on
  Product1 : Product  Inputs=**/  SaturateOnIntegerOverflow=on
  Relational Operator : RelationalOperator  RndMeth=Nearest  InputSameDT=on
  Relational Operator1 : RelationalOperator  Operator=>  RndMeth=Nearest  InputSameDT=on
  Sum : Sum  Inputs=|-+  SaturateOnIntegerOverflow=on
  Switch : Switch  Threshold=0.5  SaturateOnIntegerOverflow=on  InputSameDT=on
  Switch1 : Switch  Threshold=0.5  SaturateOnIntegerOverflow=on  InputSameDT=on
  Switch2 : Switch  Threshold=eps  SaturateOnIntegerOverflow=on  InputSameDT=on
  Switch3 : Switch  Threshold=eps  SaturateOnIntegerOverflow=on  InputSameDT=on
  To Workspace : ToWorkspace  VariableName=current_gear_ratio  SampleTime=-1
      settings: MaxDataPoints=1
  "ensure efficiency is between  0% and 100%, inclusive" : Saturate  UpperLimit=1  LowerLimit=0
  product1 : Product  SaturateOnIntegerOverflow=on
  scaled trq_out : Product  Inputs=*/  SaturateOnIntegerOverflow=on
  scaled w_out : Product  Inputs=/*  SaturateOnIntegerOverflow=on
  spd scale : Constant  Value=gb_spd_scale
  trq scale : Constant  Value=gb_trq_scale
  loss torque at input shaft (Nm) : Outport  InitialOutput=0
  wires:
  product1/1 -> Switch3/3
  Product/1 -> Switch3/1
  Switch3/1 -> Switch/1
  Constant2/1 -> Switch2/3
  [tx_eff] -> Switch3/2, Switch2/2, Switch2/1
  Switch2/1 -> Product/4
  gear_number/1 -> [gear_number]
  gear ratio/1 -> To Workspace/1, [gear_ratio]
  spd scale/1 -> scaled w_out/1
  [w_out] -> scaled w_out/2
  Sum/1 -> [one_minus_tx_eff]
  Constant1/1 -> Sum/2
  trq scale/1 -> scaled trq_out/2
  scaled trq_out/1 -> 3D discrete lookup table (sfun)/2(lookup trq (Nm))
  [T_out] -> scaled trq_out/1
  scaled w_out/1 -> 3D discrete lookup table (sfun)/1(lookup speed (rad/s))
  "ensure efficiency is between  0% and 100%, inclusive"/1 -> Sum/1, [tx_eff]
  3D discrete lookup table (sfun)/1(tx_eff) -> "ensure efficiency is between  0% and 100%, inclusive"/1
  Switch/1 -> Switch1/1
  Abs/1 -> [T_out_abs]
  Demux/1 -> Abs/1, [T_out]
  Relational Operator1/1 -> Switch1/2
  Constant3/1 -> Relational Operator1/2
  [w_out] -> Relational Operator1/1
  Constant4/1 -> Switch1/3
  Switch1/1 -> loss torque at input shaft (Nm)/1
  [gear_ratio] -> product1/2, Product/3
  [T_out_abs] -> product1/1, Product/2
  [one_minus_tx_eff] -> Product/1
  [T_out_abs] -> Product1/2
  [gear_ratio] -> Product1/3
  [one_minus_tx_eff] -> Product1/1
  Product1/1 -> Switch/3
  [T_out] -> Relational Operator/1
  Constant/1 -> Relational Operator/2
  Relational Operator/1 -> Switch/2
  [gear_number] -> 3D discrete lookup table (sfun)/3("gear_number  (e.g., 1, 2, 3)")
  Demux/2 -> [w_out]
  "output torque and speed (Nm), (rad/s)"/1 -> Demux/1

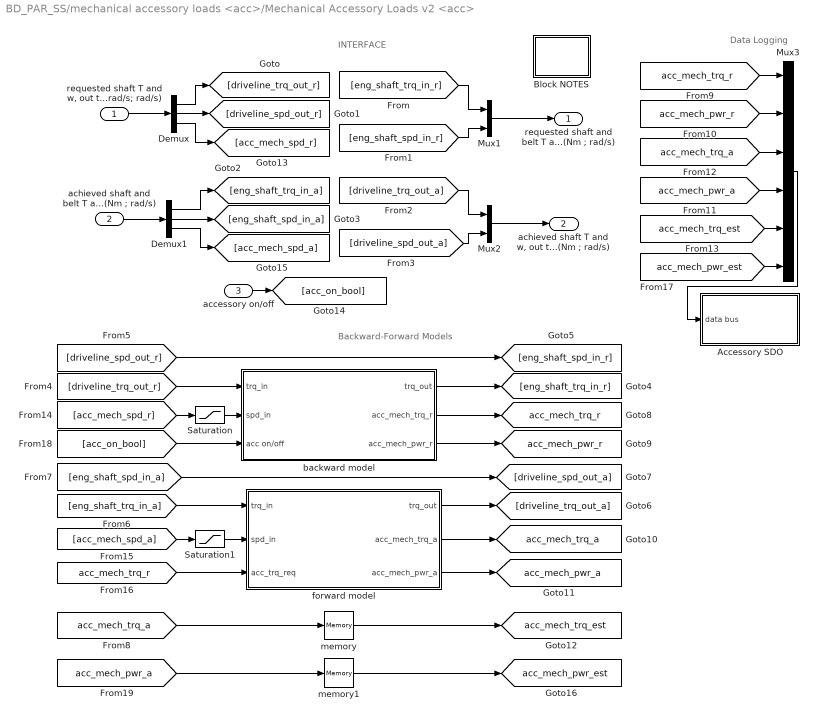
== system BD_PAR_SS/mechanical accessory loads <acc>/Mechanical Accessory Loads v2 <acc> ==
  note: Data Logging
  note: Backward-Forward Models
  note: INTERFACE
  "requested shaft T and w, out to the driveline  (Nm ; rad/s; rad/s)" : Inport
  "achieved shaft and belt T and w, in from the prime mover (Nm ; rad/s)" : Inport  Port=2
  accessory on/off : Inport  Port=3
  Accessory SDO : Subsystem
  Block NOTES : Subsystem
      mask Display: disp('Block\nNOTES')
  Demux : Demux  Outputs=3
      settings: DisplayOption=none
  Demux1 : Demux  Outputs=3
      settings: DisplayOption=none
  Mux1 : Mux  Inputs=2
  Mux2 : Mux  Inputs=2
  Mux3 : Mux  Inputs=6
  Saturation : Saturate  UpperLimit=acc_max_spd  LowerLimit=acc_min_spd
  Saturation1 : Saturate  UpperLimit=acc_max_spd  LowerLimit=acc_min_spd
  backward model : Subsystem
  forward model : Subsystem
  memory : Memory  InitialCondition=ic_mech_trq
  memory1 : Memory  InitialCondition=ic_mech_pwr
  "requested shaft and belt T and w, in from the prime mover (Nm ; rad/s)" : Outport
  "achieved shaft T and w, out to the driveline (Nm ; rad/s)" : Outport  Port=2
  tag scope: acc_mech_pwr_a=global, acc_mech_pwr_est=global, acc_mech_pwr_r=global, acc_mech_trq_a=global, acc_mech_trq_est=global, acc_mech_trq_r=global
  wires:
  [acc_mech_pwr_a] -> memory1/1
  [acc_mech_trq_a] -> memory/1
  memory1/1 -> [acc_mech_pwr_est]
  memory/1 -> [acc_mech_trq_est]
  [acc_mech_pwr_est] -> Mux3/6
  Demux/3 -> [acc_mech_spd_r]
  Demux1/3 -> [acc_mech_spd_a]
  [acc_mech_trq_r] -> forward model/3(acc_trq_req)
  Saturation/1 -> backward model/2(spd_in)
  [acc_mech_spd_r] -> Saturation/1
  Saturation1/1 -> forward model/2(spd_in)
  [acc_mech_spd_a] -> Saturation1/1
  forward model/3(acc_mech_pwr_a) -> [acc_mech_pwr_a]
  forward model/2(acc_mech_trq_a) -> [acc_mech_trq_a]
  forward model/1(trq_out) -> [driveline_trq_out_a]
  [acc_on_bool] -> backward model/3(acc on/off)
  accessory on/off/1 -> [acc_on_bool]
  [eng_shaft_trq_in_a] -> forward model/1(trq_in)
  [acc_mech_pwr_a] -> Mux3/4
  [acc_mech_trq_a] -> Mux3/3
  [eng_shaft_spd_in_a] -> [driveline_spd_out_a]
  [driveline_spd_out_r] -> [eng_shaft_spd_in_r]
  [acc_mech_trq_est] -> Mux3/5
  Mux3/1 -> Accessory SDO/1(data bus)
  [acc_mech_pwr_r] -> Mux3/2
  [acc_mech_trq_r] -> Mux3/1
  backward model/1(trq_out) -> [eng_shaft_trq_in_r]
  [driveline_trq_out_r] -> backward model/1(trq_in)
  backward model/3(acc_mech_pwr_r) -> [acc_mech_pwr_r]
  backward model/2(acc_mech_trq_r) -> [acc_mech_trq_r]
  [driveline_spd_out_a] -> Mux2/2
  [driveline_trq_out_a] -> Mux2/1
  Mux2/1 -> "achieved shaft T and w, out to the driveline (Nm ; rad/s)"/1
  [eng_shaft_spd_in_r] -> Mux1/2
  [eng_shaft_trq_in_r] -> Mux1/1
  Mux1/1 -> "requested shaft and belt T and w, in from the prime mover (Nm ; rad/s)"/1
  Demux1/2 -> [eng_shaft_spd_in_a]
  Demux1/1 -> [eng_shaft_trq_in_a]
  "achieved shaft and belt T and w, in from the prime mover (Nm ; rad/s)"/1 -> Demux1/1
  Demux/2 -> [driveline_spd_out_r]
  Demux/1 -> [driveline_trq_out_r]
  "requested shaft T and w, out to the driveline  (Nm ; rad/s; rad/s)"/1 -> Demux/1

== system BD_PAR_SS/motor/ controller <mc> par/Block NOTES ==
  note: Available torque is computed from available power by assuming that the ratio of rotor torque to input
      | (electric) power is the same for the actual/achievable situation as was computed for the request.  This
      | is mathematically equivalent to assuming that the motor/controller efficiency.  Rotor speed for the
      | actual/achievable calculations is as computed in the 'request' branch.
  note: This motor/controller model includes loss data, rotational inertia, and performance limits.

== system BD_PAR_SS/motor/ controller <mc> par/N-m drive torque per W input ==
  req'd input power (W) : Inport
  req'd rotor drive torque (Nm) : Inport  Port=2
  Block NOTES : Subsystem
      mask Display: disp('Block\nNOTES')
  Constant : Constant  Value=eps
  Constant1 : Constant  Value=0
  Constant2 : Constant  Value=inf
  Product : Product  Inputs=/*  SaturateOnIntegerOverflow=on
  Relational Operator : RelationalOperator  Operator=~=  RndMeth=Nearest  InputSameDT=on
  Sum : Sum  SaturateOnIntegerOverflow=on
  Switch : Switch  Threshold=eps  SaturateOnIntegerOverflow=on  InputSameDT=on
  Nm per W : Outport  InitialOutput=0
  wires:
  Constant2/1 -> Switch/3
  Constant1/1 -> Relational Operator/2
  req'd input power (W)/1 -> Relational Operator/1, Sum/2
  Sum/1 -> Product/1
  Switch/1 -> Nm per W/1
  Relational Operator/1 -> Switch/2
  Product/1 -> Switch/1
  req'd rotor drive torque (Nm)/1 -> Product/2
  Constant/1 -> Sum/1

== system BD_PAR_SS/motor/ controller <mc> par/documentation10 ==

== system BD_PAR_SS/motor/ controller <mc> par/effect of inertia (Nm) ==
  mc_spd_out_a : Inport
  Block NOTES : Subsystem
      mask Display: disp('Block\nNOTES')
  Constant : Constant  Value=eps
  Constant1 : Constant  Value=max(mc_max_trq)*mc_trq_scale*mc_overtrq_factor
  Constant2 : Constant  Value=gb_ratio(1)*fd_ratio/wh_radius
  Gain : Gain  Gain=mc_inertia  SaturateOnIntegerOverflow=on
  Memory : Memory
  MinMax : MinMax  Inputs=2
  Product : Product  SaturateOnIntegerOverflow=on
  Sum : Sum  SaturateOnIntegerOverflow=on
  Switch : Switch  Threshold=eps  SaturateOnIntegerOverflow=on  InputSameDT=on
  alpha : Derivative
  motor inertia as a function of total vehicle inertia (generous approximation) : Subsystem
  overall gear ratio / wh_radius : Product  Inputs=*/  SaturateOnIntegerOverflow=on
  out_1 : Outport  InitialOutput=0
  wires:
  Switch/1 -> overall gear ratio / wh_radius/2
  Constant2/1 -> Switch/3
  [veh_spd_a_rec] -> Switch/2, Sum/1
  Sum/1 -> Switch/1
  Constant/1 -> Sum/2
  motor inertia as a function of total vehicle inertia (generous approximation)/1(Out1) -> Product/2
  Memory/1 -> motor inertia as a function of total vehicle inertia (generous approximation)/1(gear ratio)
  Constant1/1 -> Product/1
  overall gear ratio / wh_radius/1 -> Memory/1
  Product/1 -> MinMax/2
  Gain/1 -> MinMax/1
  MinMax/1 -> out_1/1
  mc_spd_out_a/1 -> overall gear ratio / wh_radius/1, alpha/1
  alpha/1 -> Gain/1

== system BD_PAR_SS/motor/ controller <mc> par/enforce torque limit ==
  req'd motor torque (Nm) : Inport
  limited motor speed (rad/s) : Inport  Port=2
  Block NOTES : Subsystem
      mask Display: disp('Block\nNOTES')
  MinMax : MinMax  Inputs=2
  MinMax1 : MinMax  Function=max  Inputs=2
  Relational Operator2 : RelationalOperator  Operator=~=  RndMeth=Nearest  InputSameDT=on
  Switch : Switch  SaturateOnIntegerOverflow=on  InputSameDT=on
  To WS2 : ToWorkspace  VariableName=mc_max_trq_vec
      settings: MaxDataPoints=50000
  max gen torque : Lookup  InputValues=mc_map_spd*mc_spd_scale  Table=mc_max_gen_trq*mc_overtrq_factor*mc_trq_scale  SaturateOnIntegerOverflow=on
  max torque : Lookup  InputValues=mc_map_spd*mc_spd_scale  Table=mc_max_trq*mc_overtrq_factor*mc_trq_scale  SaturateOnIntegerOverflow=on
  limited motor torque (Nm) : Outport
  tag scope: mc_trq_limited=global
  wires:
  max gen torque/1 -> MinMax1/2
  limited motor speed (rad/s)/1 -> max gen torque/1, max torque/1
  Relational Operator2/1 -> [mc_trq_limited]
  MinMax/1 -> Switch/1
  MinMax1/1 -> Switch/3
  Switch/1 -> limited motor torque (Nm)/1, Relational Operator2/2
  req'd motor torque (Nm)/1 -> MinMax/1, MinMax1/1, Switch/2, Relational Operator2/1
  max torque/1 -> MinMax/2, To WS2/1

== system BD_PAR_SS/motor/ controller <mc> par/mc tmp ==
  Qmc_gen : Inport
  veh spd : Inport  Port=2
  key ON? : Inport  Port=3
  Enable : EnablePort  StatesWhenEnabling=reset
  1/mcp : Gain  Gain=1/(mc_mass*mc_cp)  SaturateOnIntegerOverflow=on
  >=0 : Saturate  UpperLimit=Inf  LowerLimit=0
  ">=0 " : Saturate  UpperLimit=Inf  LowerLimit=0
  Block NOTES : Subsystem
      mask Display: disp('Block\nNOTES')
  Mux10 : Mux  Inputs=2
  Mux9 : Mux  Inputs=2
  Qa : Fcn  Expr=u(1)*(mc_sarea*mc_trq_scale*mc_spd_scale)*u(2)
  Qc1 : Sum  Inputs=-+  SaturateOnIntegerOverflow=on
  Qnet : Sum  Inputs=+++  SaturateOnIntegerOverflow=on
  Qp2a,v7 : Fcn  Expr=amb_tmp-u(1)
  Qr : Fcn  Expr=0.9*(5.67e-8)*(mc_sarea*mc_trq_scale*mc_spd_scale)*((amb_tmp+273)^4 - (u(1)+273)^4)
  Tmc3 : Integrator  InitialCondition=mc_init_tmp
  Va/Vv : Gain  Gain=0.5  SaturateOnIntegerOverflow=on
  ha : Fcn  Expr=6 + 6*((abs(u(2))/1000))^0.25 + 60*(abs(u(1))/30)^0.63
  mc coolant : Subsystem  TreatAsAtomicUnit=on
  Tmc : Outport  InitialOutput=0
  Qmc_clt : Outport  Port=2  OutputWhenDisabled=reset  InitialOutput=0
  wires:
  Qnet/1 -> Qc1/2, mc coolant/2("Qmc ")
  Qc1/1 -> 1/mcp/1
  1/mcp/1 -> Tmc3/1
  Tmc3/1 -> Qp2a,v7/1, Qr/1, Tmc/1, mc coolant/1(Tcl)
  mc coolant/1(Qmc_clt) -> Qc1/1, >=0/1
  >=0/1 -> Qmc_clt/1
  key ON?/1 -> mc coolant/Enable
  veh spd/1 -> Va/Vv/1
  Qa/1 -> Qnet/2
  ">=0 "/1 -> Qnet/1
  Qmc_gen/1 -> ">=0 "/1
  Qr/1 -> Qnet/3
  Qp2a,v7/1 -> Mux10/2, Mux9/2
  ha/1 -> Mux10/1
  Va/Vv/1 -> Mux9/1
  Mux9/1 -> ha/1
  Mux10/1 -> Qa/1

== system BD_PAR_SS/motor/ controller <mc> par/motor controller logic interface ==
  w_mc_out_r : Inport
  P_mc_in_1lim : Inport  Port=2
  P_mc_in_r : Outport  InitialOutput=0
  tag scope: P_mc_in_1lim=global, w_mc_out_r=global
  wires:
  [P_mc_in_r] -> P_mc_in_r/1
  w_mc_out_r/1 -> [w_mc_out_r]
  P_mc_in_1lim/1 -> [P_mc_in_1lim]
